simulink model "Closed_Loop_System_app1"  (R2018b)
settings: Solver=VariableStepAuto  StartTime=0.0  StopTime=10  RelTol=1e-3
StopFcn:
  | close all
  | pos_n=pos.signals.values;
  | t=pos.time;
  | pos_rn=pos_r.signals.values;
  | 
  | for i=1:6
  | figure(i)
  |     plot(t,pos_n(:,i),'b-','LineWidth',2)
  |     hold on
  |     plot(t,pos_rn(:,i),'r--','LineWidth',2)
  |     xlabel('time (s)')
  |     ylabel(['X',num2str(i)])
  |     legend('actual','desired')
  |     grid
  | end
  | figure(7)
  | plot3(pos_n(:,1),pos_n(:,2),pos_n(:,3),'b-','LineWidth',2)
  | hold on
  | plot3(pos_rn(:,1),pos_rn(:,2),pos_rn(:,3),'r--','LineWidth',2)
  |     xlabel('time (s)')
  |     ylabel(['X',num2str(i)])
  |     grid
  |     legend('actual End eff. trajectory','desired End eff. trajectory')
values from neighbouring files (symbols this model uses):
  pos = [loc;orientation]    [Direct_Kinematic.m]
settings Model: Creator=HJokar  LastModifiedBy=HJokar

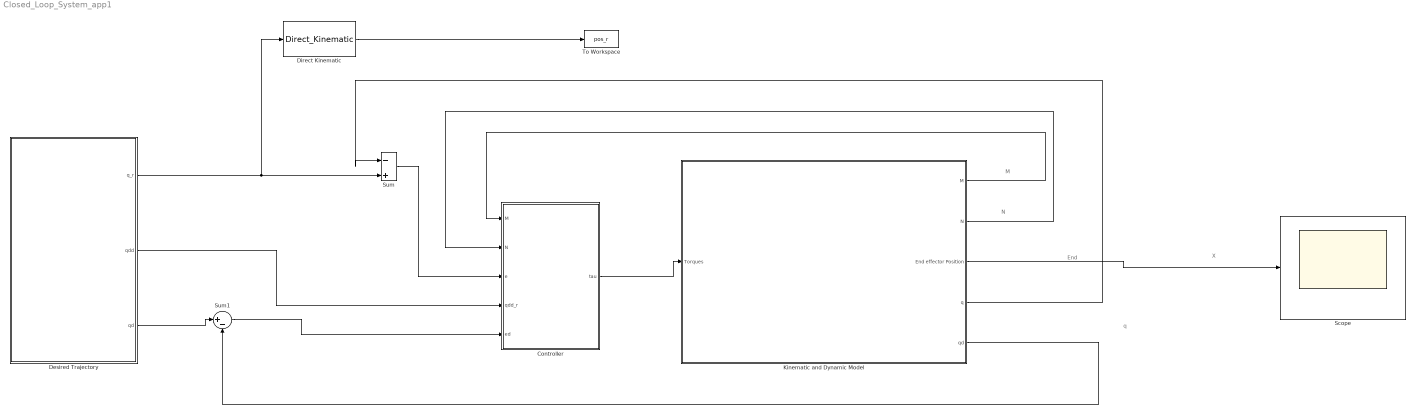
== system Closed_Loop_System_app1 ==
  note: X
  note: End
  note: N
  note: M
  note: q
  Controller : MATLAB Function  TreatAsAtomicUnit=on
  Desired Trajectory : Subsystem
  Direct Kinematic : MATLABFcn  MATLABFcn=Direct_Kinematic  OutputSignalType=real
  Kinematic and Dynamic Model : Subsystem
      mask Display: image('robotfig.png');
  Scope : Scope
  Sum : Sum  Inputs=|-+
  Sum1 : Sum  Inputs=|+-
  To Workspace : ToWorkspace  VariableName=pos_r  SaveFormat=Structure With Time  SampleTime=-1
  wires:
  Kinematic and Dynamic Model/5(qd) -> Sum1/2
  Sum/1 -> Controller/3(e)
  Sum1/1 -> Controller/5(ed)
  Kinematic and Dynamic Model/1(M) -> Controller/1(M)
  Kinematic and Dynamic Model/2(N) -> Controller/2(N)
  Kinematic and Dynamic Model/3(End effector Position) -> Scope/1
  Controller/1(tau) -> Kinematic and Dynamic Model/1(Torques)
  Desired Trajectory/1(q_r) -> Direct Kinematic/1, Sum/2
  Desired Trajectory/3(qd) -> Sum1/1
  Desired Trajectory/2(qdd) -> Controller/4(qdd_r)
  Kinematic and Dynamic Model/4(q) -> Sum/1
  Direct Kinematic/1 -> To Workspace/1

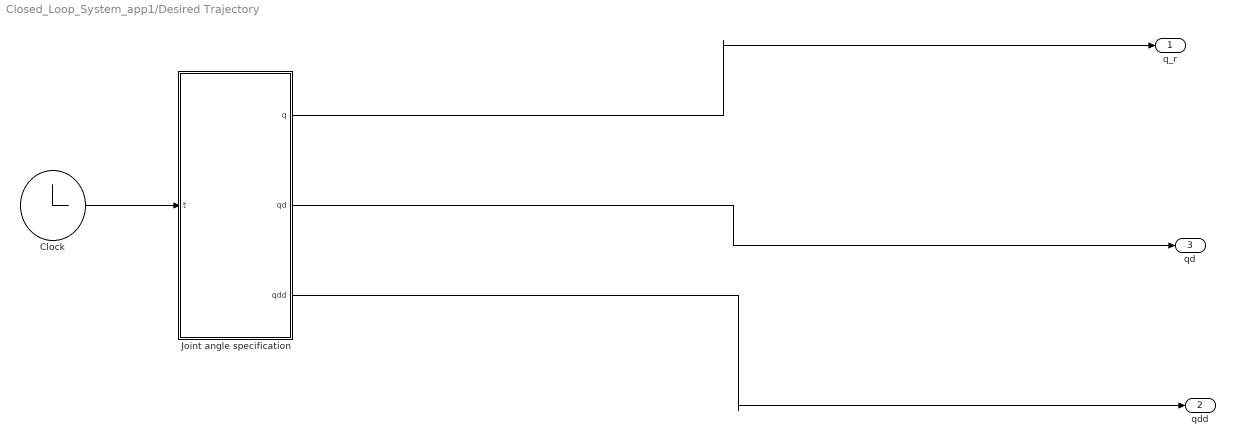
== system Closed_Loop_System_app1/Desired Trajectory ==
  Clock : Clock
  Joint angle specification : MATLAB Function  TreatAsAtomicUnit=on
  q_r : Outport
  qdd : Outport  Port=2
  qd : Outport  Port=3
  wires:
  Clock/1 -> Joint angle specification/1(t)
  Joint angle specification/3(qdd) -> qdd/1
  Joint angle specification/1(q) -> q_r/1
  Joint angle specification/2(qd) -> qd/1

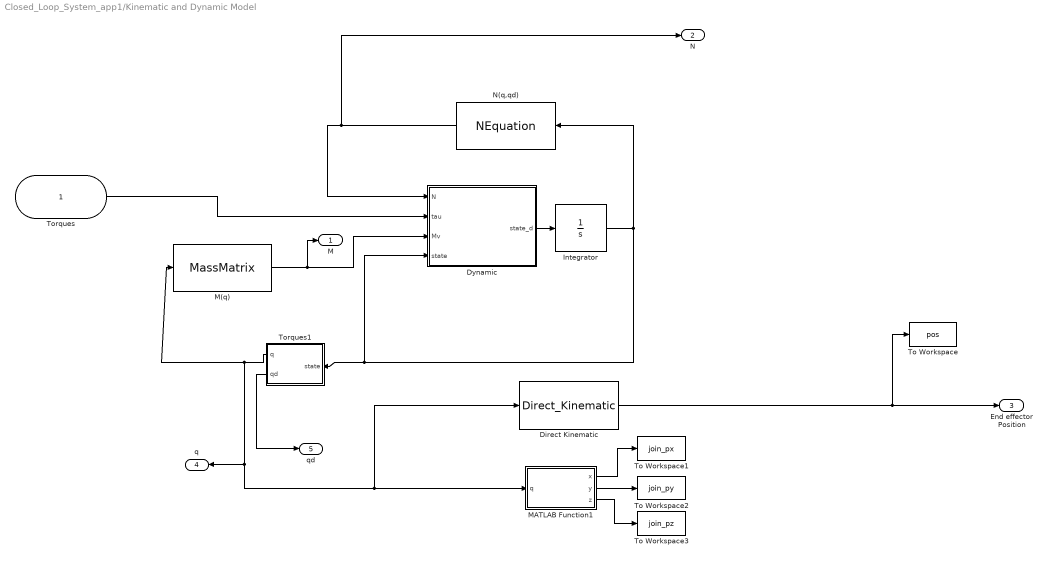
== system Closed_Loop_System_app1/Kinematic and Dynamic Model ==
  Torques : Inport
  Direct Kinematic : MATLABFcn  MATLABFcn=Direct_Kinematic  OutputSignalType=real
  Dynamic : MATLAB Function  TreatAsAtomicUnit=on
  Integrator : Integrator  InitialCondition=zeros(14,1)
  M(q) : MATLABFcn  MATLABFcn=MassMatrix  OutputSignalType=real
  MATLAB Function1 : MATLAB Function  TreatAsAtomicUnit=on
  N(q,qd) : MATLABFcn  MATLABFcn=NEquation  OutputSignalType=real
  To Workspace : ToWorkspace  VariableName=pos  SaveFormat=Structure With Time  SampleTime=-1
  To Workspace1 : ToWorkspace  VariableName=join_px  SaveFormat=Structure With Time  SampleTime=-1
  To Workspace2 : ToWorkspace  VariableName=join_py  SaveFormat=Structure With Time  SampleTime=-1
  To Workspace3 : ToWorkspace  VariableName=join_pz  SaveFormat=Structure With Time  SampleTime=-1
  Torques1 : MATLAB Function  TreatAsAtomicUnit=on
  M : Outport
  N : Outport  Port=2
  End effector Position : Outport  Port=3
  q : Outport  Port=4
  qd : Outport  Port=5
  wires:
  MATLAB Function1/3(z) -> To Workspace3/1
  M(q)/1 -> M/1, Dynamic/3(Mv)
  Torques/1 -> Dynamic/2(tau)
  Torques1/1(q) -> MATLAB Function1/1(q), Direct Kinematic/1, q/1, M(q)/1
  Direct Kinematic/1 -> To Workspace/1, End effector Position/1
  Dynamic/1(state_d) -> Integrator/1
  MATLAB Function1/1(x) -> To Workspace1/1
  Integrator/1 -> N(q,qd)/1, Dynamic/4(state), Torques1/1(state)
  MATLAB Function1/2(y) -> To Workspace2/1
  Torques1/2(qd) -> qd/1
  N(q,qd)/1 -> Dynamic/1(N), N/1

== matlab function Closed_Loop_System_app1/Kinematic and Dynamic Model/Dynamic ==
  data: N input; state_d output; tau input; Mv input; state input
function  state_d= Dynamic_model(N,tau,Mv,state)
nL=7;
state_d=zeros(2*nL,1);
q=state(1:nL);
qd=state(nL+1:2*nL);
M=reshape(Mv,[nL,nL]);
%=============== Dynamic ====================
qdd=M^(-1)*(tau-N);
state_d(1:nL)=qd;
state_d(nL+1:2*nL)=qdd;
end

== matlab function Closed_Loop_System_app1/Kinematic and Dynamic Model/Torques1 ==
  data: q output; state input; qd output
function [q,qd ] = fcn(state)
nL=7;
q=state(1:nL);
qd=state(nL+1:2*nL);

== matlab function Closed_Loop_System_app1/Kinematic and Dynamic Model/MATLAB Function1 ==
  data: q input; x output; y output; z output
function [x,y,z]=Frame_origin(q)

nL=7;
d=[317*cos(asin(81/317)) 194.5 400 168.5 400 136.3 134.75]'*1e-3;
a=[0 81 0 0 0 0 0]'*1e-3; 
alpha=[0 -pi/2 -pi/2 -pi/2 pi/2 pi/2 -pi/2]';
teta=q;
teta(2)=teta(2)-pi/2;
Ti_im={zeros(4,4),zeros(4,4),zeros(4,4),zeros(4,4),zeros(4,4),zeros(4,4),zeros(4,4)};
Ti=Ti_im;
for i = 1:nL
    Ti_im{i} =[ cos(teta(i)) -sin(teta(i)) 0 a(i);
        sin(teta(i))*cos(alpha(i)) cos(teta(i))*cos(alpha(i)) -sin(alpha(i)) -sin(alpha(i))*d(i);
        sin(teta(i))*sin(alpha(i)) cos(teta(i))*sin(alpha(i)) cos(alpha(i)) cos(alpha(i))*d(i);
        0 0 0 1];
end
% 0_T_i
for i = 1:nL
    if i==1
        Ti{i}=Ti_im{i};
        
    else
        Ti{i}=Ti{i-1}*Ti_im{i};
    end
end
% Robot Configuration:

x=[0,Ti{1}(1,4) Ti{2}(1,4) Ti{3}(1,4) Ti{4}(1,4) Ti{5}(1,4) Ti{6}(1,4) Ti{7}(1,4)]';
y=[0,Ti{1}(2,4) Ti{2}(2,4) Ti{3}(2,4) Ti{4}(2,4) Ti{5}(2,4) Ti{6}(2,4) Ti{7}(2,4)]';
z=[0,Ti{1}(3,4) Ti{2}(3,4) Ti{3}(3,4) Ti{4}(3,4) Ti{5}(3,4) Ti{6}(3,4) Ti{7}(3,4)]';
end

== matlab function Closed_Loop_System_app1/Controller ==
  data: M input; N input; e input; qdd_r input; ed input; tau output
function tau = Controller(M,N,e,qdd_r,ed)
tau=zeros(7,1);


Kp=100*eye(7);
Kd=100*eye(7);

nL=7;


M=reshape(M,[nL,nL]);
u=-Kp*e-Kd*ed;
tau=M*(qdd_r-u)+N;

== matlab function Closed_Loop_System_app1/Desired Trajectory/Joint angle specification ==
  data: t input; q output; qd output; qdd output
function [q,qd,qdd] = fcn(t)
q=zeros(7,1);
q(1)=pi/2;
q(2)=-pi/2;
q(3)=pi/4;
q(4)=pi/4;
q(5)=pi/4;
q(6)=pi/4;
q(7)=pi/4;


qd=zeros(7,1);
qd(1)=0;
qd(2)=0;
qd(3)=0;
qd(4)=0;
qd(5)=0;
qd(6)=0;
qd(7)=0;

qdd=zeros(7,1);
qdd(1)=0;
qdd(2)=0;
qdd(3)=0;
qdd(4)=0;
qdd(5)=0;
qdd(6)=0;
qdd(7)=0;
